simulink model "simulacaoOrientacaoESC_SIAC"  (R2015a)
settings: Solver=ode4  StartTime=0.0  StopTime=30  FixedStep=0.0001  RelTol=1e-3
values from neighbouring files (symbols this model uses):
  ampSenoide = 15    [simuOrientacaoESC.m]
  freqSenoide = 1.5*2*pi    (= 9.42477796077)    [simuOrientacaoESC.m]
  K = 1    [simuOrientacaoESC.m]
  Kp = 10    [simuOrientacaoESC.m]
undefined symbols (not defined in the file or in its folder): xL0
settings Model: Creator=Jean  LastModifiedBy=Jean

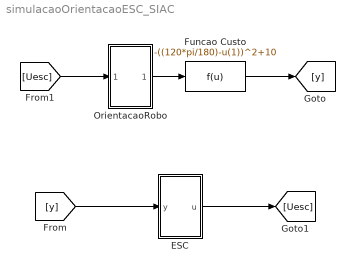
== system simulacaoOrientacaoESC_SIAC ==
  ESC : Subsystem
  Funcao Custo : Fcn  Expr=-((120*pi/180)-u(1))^2+10
  "OrientacaoRobo " : Subsystem
  wires:
  [Uesc] -> "OrientacaoRobo "/1(In1)
  [y] -> ESC/1(y)
  ESC/1(u) -> [Uesc]
  "OrientacaoRobo "/1(Out1) -> Funcao Custo/1
  Funcao Custo/1 -> [y]

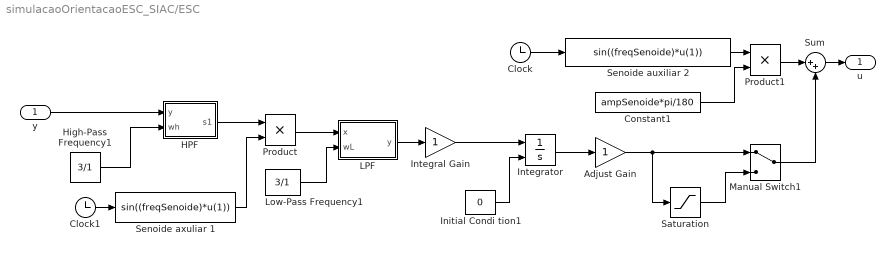
== system simulacaoOrientacaoESC_SIAC/ESC ==
  y : Inport
  Adjust Gain : Gain
  Clock : Clock
  Clock1 : Clock
  Constant1 : Constant  Value=ampSenoide*pi/180  SampleTime=Inf
  HPF : Subsystem
  High-Pass Frequency1 : Constant  Value=3/1  SampleTime=Inf
  Initial Condi tion1 : Constant  Value=0  SampleTime=Inf
  Integral Gain : Gain
  Integrator : Integrator  InitialConditionSource=external
  LPF : Subsystem
  Low-Pass Frequency1 : Constant  Value=3/1  SampleTime=Inf
  Manual Switch1 : ManualSwitch
  Product : Product
  Product1 : Product
  Saturation : Saturate  UpperLimit=100  LowerLimit=-100
  Senoide auxiliar 2 : Fcn  Expr=sin((freqSenoide)*u(1))
  "Senoide axuliar 1 " : Fcn  Expr=sin((freqSenoide)*u(1))
  Sum : Sum  Inputs=|++
  u : Outport
  wires:
  Sum/1 -> u/1
  Product1/1 -> Sum/1
  Senoide auxiliar 2/1 -> Product1/1
  Integrator/1 -> Adjust Gain/1
  y/1 -> HPF/1(y)
  Manual Switch1/1 -> Sum/2
  Clock/1 -> Senoide auxiliar 2/1
  Clock1/1 -> "Senoide axuliar 1 "/1
  HPF/1(s1) -> Product/1
  Adjust Gain/1 -> Manual Switch1/1, Saturation/1
  LPF/1(y) -> Integral Gain/1
  Integral Gain/1 -> Integrator/1
  Saturation/1 -> Manual Switch1/2
  Product/1 -> LPF/1(x)
  High-Pass Frequency1/1 -> HPF/2(wh)
  "Senoide axuliar 1 "/1 -> Product/2
  Low-Pass Frequency1/1 -> LPF/2(wL)
  Initial Condi tion1/1 -> Integrator/2
  Constant1/1 -> Product1/2

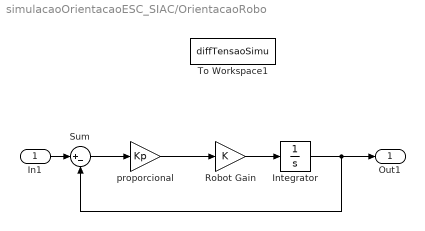
== system simulacaoOrientacaoESC_SIAC/OrientacaoRobo  ==
  In1 : Inport
  Integrator : Integrator
  Robot Gain : Gain  Gain=K
  Sum : Sum  Inputs=|+-
  To Workspace1 : ToWorkspace  VariableName=diffTensaoSimu  SaveFormat=Structure With Time  SampleTime=-1
  "proporcional " : Gain  Gain=Kp
  Out1 : Outport
  wires:
  Robot Gain/1 -> Integrator/1
  Integrator/1 -> Out1/1, Sum/2
  In1/1 -> Sum/1
  "proporcional "/1 -> Robot Gain/1
  Sum/1 -> "proporcional "/1

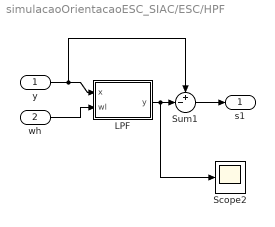
== system simulacaoOrientacaoESC_SIAC/ESC/HPF ==
  y : Inport
  wh : Inport  Port=2
  LPF : Subsystem
  Scope2 : Scope
      settings: YMin=0.6  YMax=1.125  SaveName=ScopeData5
  Sum1 : Sum  Inputs=+-|
  s1 : Outport
  wires:
  LPF/1(y) -> Sum1/2, Scope2/1
  wh/1 -> LPF/2(wl)
  Sum1/1 -> s1/1
  y/1 -> Sum1/1, LPF/1(x)

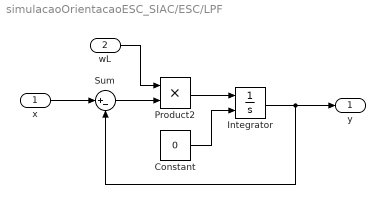
== system simulacaoOrientacaoESC_SIAC/ESC/LPF ==
  x : Inport
  wL : Inport  Port=2
  Constant : Constant  Value=0
  Integrator : Integrator  InitialConditionSource=external  InitialCondition=xL0
  Product2 : Product
  Sum : Sum  Inputs=|+-
  y : Outport
  wires:
  Constant/1 -> Integrator/2
  x/1 -> Sum/1
  Sum/1 -> Product2/2
  Product2/1 -> Integrator/1
  Integrator/1 -> y/1, Sum/2
  wL/1 -> Product2/1

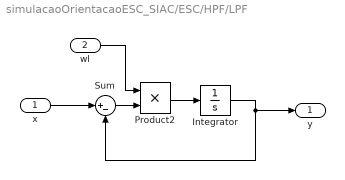
== system simulacaoOrientacaoESC_SIAC/ESC/HPF/LPF ==
  x : Inport
  wl : Inport  Port=2
  Integrator : Integrator
  Product2 : Product
  Sum : Sum  Inputs=|+-
  y : Outport
  wires:
  wl/1 -> Product2/1
  Integrator/1 -> y/1, Sum/2
  Product2/1 -> Integrator/1
  Sum/1 -> Product2/2
  x/1 -> Sum/1
